simulink model "line_followzr"  (R2020a)
settings: Solver=FixedStepAuto  StartTime=0.0  StopTime=inf  RelTol=1e-3  EnableMultiTasking=on
libraries: arduinolib x8, simulink x4
settings Model: SILPILModeSetting=veronly  ExtModeTrigDuration=2  Creator=kelko  LastModifiedBy=kelko
settings OptimizationCC: EnhancedBackFolding=on  PassReuseOutputArgsAs=Individual arguments  ZeroExternalMemoryAtStartup=off  ZeroInternalMemoryAtStartup=off  MaxStackSize=64  OptimizeBlockOrder=speed  DifferentSizesBufferReuse=on  OptimizationCustomize=off  EfficientTunableParamExpr=on
settings DebuggingCC: ParameterTunabilityLossMsg=error
settings HardwareCC: ProdBitPerInt=16  ProdBitPerPointer=16  ProdBitPerSizeT=16  ProdBitPerPtrDiffT=16  ProdLargestAtomicFloat=None  ProdWordSize=8  ProdHWDeviceType=Atmel->AVR
settings SFSimCC: MATLABDynamicMemAlloc=off
settings RTWCC: SystemTargetFile=ert.tlc  HardwareBoard=Arduino Uno  TLCOptions=-aInlineSetEventsForThisBaseRateFcn=TLC_FALSE -aSuppressMultiTaskScheduler=TLC_FALSE -aRateBasedStepFcn=1  TemplateMakefile=ert_default_tmf  Toolchain=Arduino AVR  BuildConfiguration=Faster Runs
settings CodeAppCC: ForceParamTrailComments=on  IgnoreCustomStorageClasses=off  OperatorAnnotations=on  SimulinkDataObjDesc=on  SFDataObjDesc=on  InsertBlockDesc=on
settings ERTTargetCC: SupportContinuousTime=on  SupportVariableSizeSignals=on  ExtModeStaticAllocSize=250

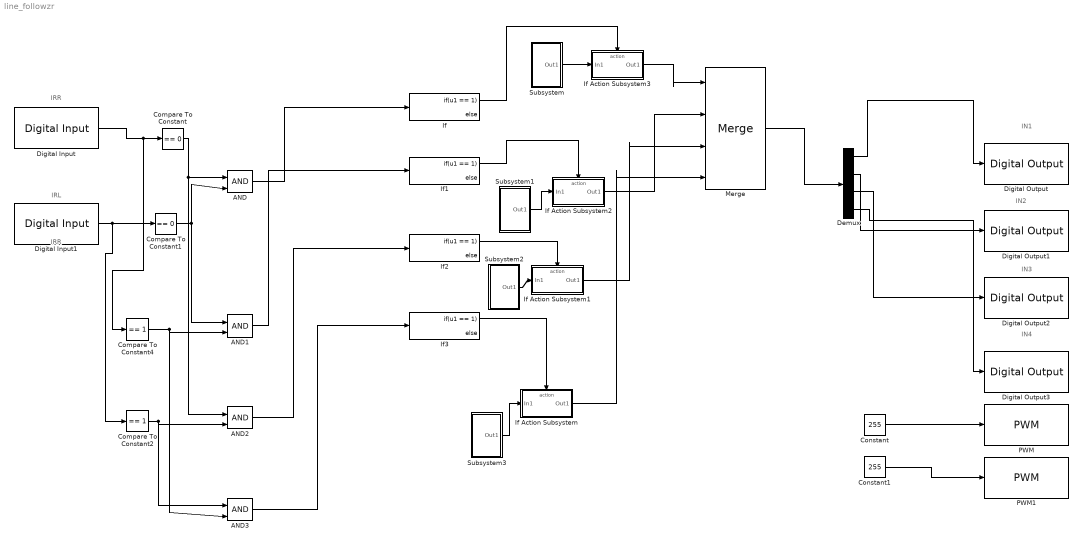
== system line_followzr ==
  note: IN1
  note: IN2
  note: IN3
  note: IN4
  note: IRR
  note: IRL
  note: IRR
  AND{,1..3} (4 alike) : Logic  IconShape=distinctive  AllPortsSameDT=off  OutDataTypeStr=boolean
  Compare To Constant : simulink/Logic and Bit Operations/Compare To Constant  relop===  const=0  OutDataTypeStr=boolean
  Compare To Constant1 : simulink/Logic and Bit Operations/Compare To Constant  relop===  const=0  OutDataTypeStr=boolean
  Compare To Constant2 : simulink/Logic and Bit Operations/Compare To Constant  relop===  const=1  OutDataTypeStr=boolean
  Compare To Constant4 : simulink/Logic and Bit Operations/Compare To Constant  relop===  const=1  OutDataTypeStr=boolean
  Constant : Constant  Value=255
  Constant1 : Constant  Value=255
  Demux : Demux
  Digital Input : arduinolib/Digital Input  pinNumber=2  Direction=input  SampleTime=0.001  blockPlatform=arduino
  Digital Input1 : arduinolib/Digital Input  pinNumber=3  Direction=input  SampleTime=0.001  blockPlatform=arduino
  Digital Output : arduinolib/Digital Output  pinNumber=4  Direction=output  blockPlatform=arduino
  Digital Output1 : arduinolib/Digital Output  pinNumber=5  Direction=output  blockPlatform=arduino
  Digital Output2 : arduinolib/Digital Output  pinNumber=6  Direction=output  blockPlatform=arduino
  Digital Output3 : arduinolib/Digital Output  pinNumber=7  Direction=output  blockPlatform=arduino
  If{,1..3} (4 alike) : If  IfExpression=u1 == 1
  If Action Subsystem : Subsystem  TreatAsAtomicUnit=on
  If Action Subsystem1 : Subsystem  TreatAsAtomicUnit=on
  If Action Subsystem2 : Subsystem  TreatAsAtomicUnit=on
  If Action Subsystem3 : Subsystem  TreatAsAtomicUnit=on
  Merge : Merge  Inputs=4
  PWM : arduinolib/PWM  pinNumber=9  frequencyType=Default  desiredFrequency=490.2  achievableFrequency=490.2
  PWM1 : arduinolib/PWM  pinNumber=10  frequencyType=Default  desiredFrequency=490.2  achievableFrequency=490.2
  Subsystem : Subsystem
  Subsystem1 : Subsystem
  Subsystem2 : Subsystem
  Subsystem3 : Subsystem
  wires:
  Compare To Constant2/1 -> AND3/1, AND2/2
  Compare To Constant1/1 -> AND1/1, AND/2
  Digital Input/1 -> Compare To Constant4/1, Compare To Constant/1
  Compare To Constant4/1 -> AND3/2, AND1/2
  Digital Input1/1 -> Compare To Constant2/1, Compare To Constant1/1
  Compare To Constant/1 -> AND2/1, AND/1
  AND/1 -> If/1
  AND1/1 -> If1/1
  AND2/1 -> If2/1
  AND3/1 -> If3/1
  If3/1 -> If Action Subsystem/Action
  Subsystem3/1(Out1) -> If Action Subsystem/1(In1)
  If2/1 -> If Action Subsystem1/Action
  Subsystem2/1(Out1) -> If Action Subsystem1/1(In1)
  If/1 -> If Action Subsystem3/Action
  If1/1 -> If Action Subsystem2/Action
  Subsystem1/1(Out1) -> If Action Subsystem2/1(In1)
  Subsystem/1(Out1) -> If Action Subsystem3/1(In1)
  If Action Subsystem3/1(Out1) -> Merge/1
  If Action Subsystem2/1(Out1) -> Merge/2
  If Action Subsystem1/1(Out1) -> Merge/3
  If Action Subsystem/1(Out1) -> Merge/4
  Merge/1 -> Demux/1
  Constant/1 -> PWM/1
  Constant1/1 -> PWM1/1
  Demux/1 -> Digital Output/1
  Demux/2 -> Digital Output1/1
  Demux/3 -> Digital Output2/1
  Demux/4 -> Digital Output3/1

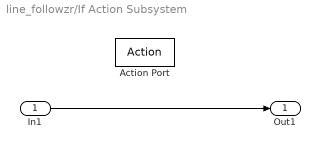
== system line_followzr/If Action Subsystem ==
  In1 : Inport
  Action Port : ActionPort  ActionPortLabel=if(u1 == 1)
  Out1 : Outport
  wires:
  In1/1 -> Out1/1

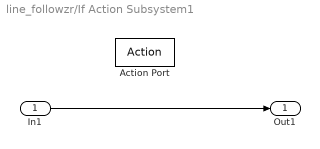
== system line_followzr/If Action Subsystem1 ==
  In1 : Inport
  Action Port : ActionPort  ActionPortLabel=if(u1 == 1)
  Out1 : Outport
  wires:
  In1/1 -> Out1/1

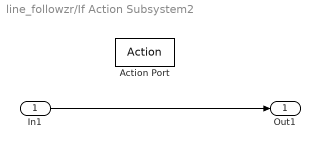
== system line_followzr/If Action Subsystem2 ==
  In1 : Inport
  Action Port : ActionPort  ActionPortLabel=if(u1 == 1)
  Out1 : Outport
  wires:
  In1/1 -> Out1/1

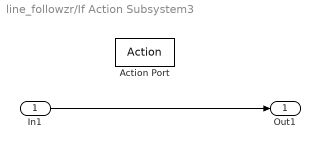
== system line_followzr/If Action Subsystem3 ==
  In1 : Inport
  Action Port : ActionPort  ActionPortLabel=if(u1 == 1)
  Out1 : Outport
  wires:
  In1/1 -> Out1/1

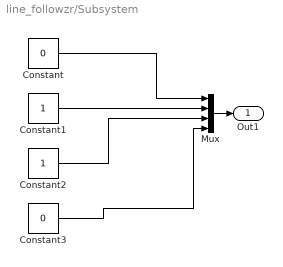
== system line_followzr/Subsystem ==
  Constant : Constant  Value=0
  Constant1 : Constant
  Constant2 : Constant
  Constant3 : Constant  Value=0
  Mux : Mux
  Out1 : Outport
  wires:
  Constant/1 -> Mux/1
  Mux/1 -> Out1/1
  Constant2/1 -> Mux/3
  Constant1/1 -> Mux/2
  Constant3/1 -> Mux/4

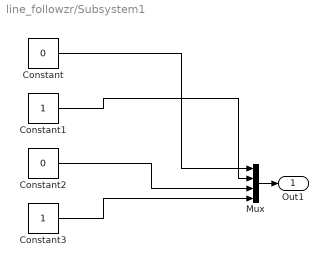
== system line_followzr/Subsystem1 ==
  Constant : Constant  Value=0
  Constant1 : Constant
  Constant2 : Constant  Value=0
  Constant3 : Constant
  Mux : Mux
  Out1 : Outport
  wires:
  Mux/1 -> Out1/1
  Constant1/1 -> Mux/2
  Constant/1 -> Mux/1
  Constant3/1 -> Mux/4
  Constant2/1 -> Mux/3

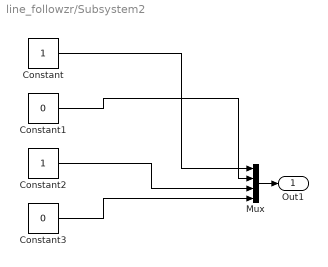
== system line_followzr/Subsystem2 ==
  Constant : Constant
  Constant1 : Constant  Value=0
  Constant2 : Constant
  Constant3 : Constant  Value=0
  Mux : Mux
  Out1 : Outport
  wires:
  Constant2/1 -> Mux/3
  Constant3/1 -> Mux/4
  Constant/1 -> Mux/1
  Constant1/1 -> Mux/2
  Mux/1 -> Out1/1

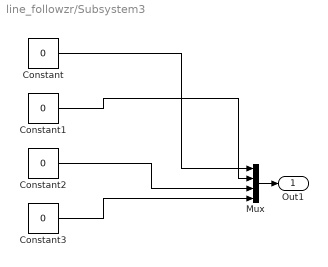
== system line_followzr/Subsystem3 ==
  Constant{,1..3} (4 alike) : Constant  Value=0
  Mux : Mux
  Out1 : Outport
  wires:
  Mux/1 -> Out1/1
  Constant1/1 -> Mux/2
  Constant/1 -> Mux/1
  Constant3/1 -> Mux/4
  Constant2/1 -> Mux/3
